simulink model "modelident_r2"  (R2013a)
settings: Solver=ode3  StartTime=0.0  StopTime=50  FixedStep=.001  RelTol=1e-3
settings Model: Creator=Chris D'Angelo  LastModifiedBy=Chris D'Angelo

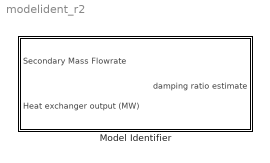
== system modelident_r2 ==
  Model Identifier : Subsystem

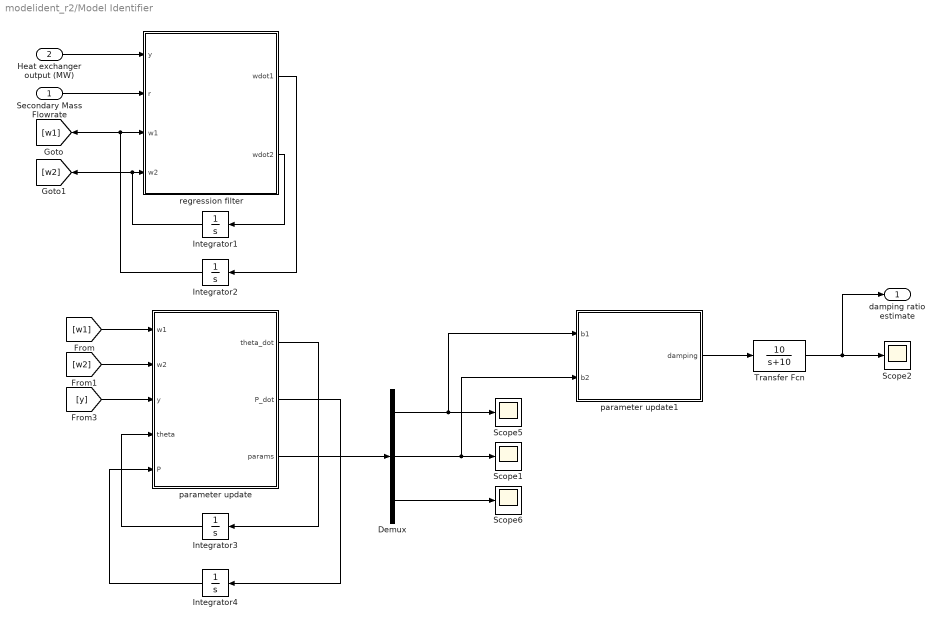
== system modelident_r2/Model Identifier ==
  Secondary Mass Flowrate : Inport
  Heat exchanger output (MW) : Inport  Port=2
  Demux : Demux  Outputs=3
  Integrator1 : Integrator  InitialCondition=0.5*ones(2,1)
  Integrator2 : Integrator  InitialCondition=0.5*ones(2,1)
  Integrator3 : Integrator  InitialCondition=5*ones(4,1)
  Integrator4 : Integrator  InitialCondition=10*eye(4)
  Scope{1..2,5..6} (4 alike) : Scope
      Scope1 settings: TimeRange=50  YMax=2
      Scope2 settings: SaveName=ScopeData2
      Scope5 settings: TimeRange=50  YMin=1.83  YMax=1.93  SaveName=ScopeData5
      Scope6 settings: TimeRange=50  YMax=2  SaveName=ScopeData6
  Transfer Fcn : TransferFcn  Numerator=[10]  Denominator=[1 10]
  parameter update : MATLAB Function  TreatAsAtomicUnit=on
  parameter update1 : MATLAB Function  TreatAsAtomicUnit=on
  regression filter : MATLAB Function  TreatAsAtomicUnit=on
  damping ratio estimate : Outport
  wires:
  parameter update1/1(damping) -> Transfer Fcn/1
  regression filter/2(wdot2) -> Integrator1/1
  regression filter/1(wdot1) -> Integrator2/1
  Integrator1/1 -> [w2], regression filter/4(w2)
  Integrator2/1 -> [w1], regression filter/3(w1)
  parameter update/1(theta_dot) -> Integrator3/1
  Integrator3/1 -> parameter update/4(theta)
  parameter update/3(params) -> Demux/1
  Demux/2 -> parameter update1/2(b2), Scope1/1
  Demux/1 -> parameter update1/1(b1), Scope5/1
  Demux/3 -> Scope6/1
  parameter update/2(P_dot) -> Integrator4/1
  Integrator4/1 -> parameter update/5(P)
  [w1] -> parameter update/1(w1)
  [w2] -> parameter update/2(w2)
  Heat exchanger output (MW)/1 -> regression filter/1(y)
  [y] -> parameter update/3(y)
  Secondary Mass Flowrate/1 -> regression filter/2(r)
  Transfer Fcn/1 -> damping ratio estimate/1, Scope2/1

== matlab function modelident_r2/Model Identifier/regression filter ==
  data: y input; r input; w1 input; w2 input; wdot1 output; wdot2 output
function [wdot1,wdot2] = filter(y,r,w1,w2)

Lambda = [0 1;-4 -4]; %Hurwitz filter in controllable canonical form
bL = [0;1];

wdot1 = Lambda*w1 + bL*r; %filtered plant input
wdot2 = Lambda*w2 + bL*y; %filtered plant output

== matlab function modelident_r2/Model Identifier/parameter update ==
  data: w1 input; theta_dot output; P_dot output; w2 input; y input; theta input; params output; P input
function [theta_dot,P_dot,params] = parameterupdate(w1,w2,y,theta,P)
%#codegen

%w1 is from input, w2 is from output (y_plant)

g = .5;
w = [w2;w1];
yi = theta'*w;
e = yi-y;
theta_dot = -g*P*w*e * ((1 + 1*w'*P*w)^-1);
P_dot = g*5*P - g*P*w*w'*P;

params = [4;4;0] - [theta(1);theta(2);theta(3)]  ;

== matlab function modelident_r2/Model Identifier/parameter update1 ==
  data: b1 input; damping output; b2 input
function damping = dampingratio(b1,b2)

if b1<0
    b1 = sqrt(abs(b1));
else
    b1 = sqrt(b1);
end

damping = 0.5*1/b1 * b2;
